simulink model "untitled"  (R2022b)
settings: Solver=VariableStepAuto  StartTime=0.0  StopTime=10.0  RelTol=1e-3
undefined symbols (not defined in the file): F, g, J, M, mass, quadrotor
libraries: slpidlib x4, simulink x2, matrix_library x1
settings Model: Creator=Musta  LastModifiedBy=Musta

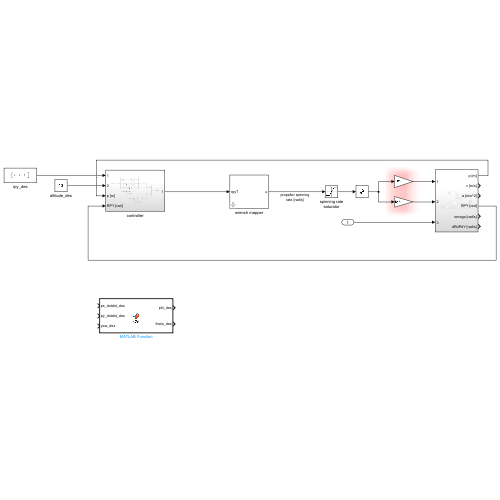
[thumbnail: Simulink's stored preview of the top-level diagram]
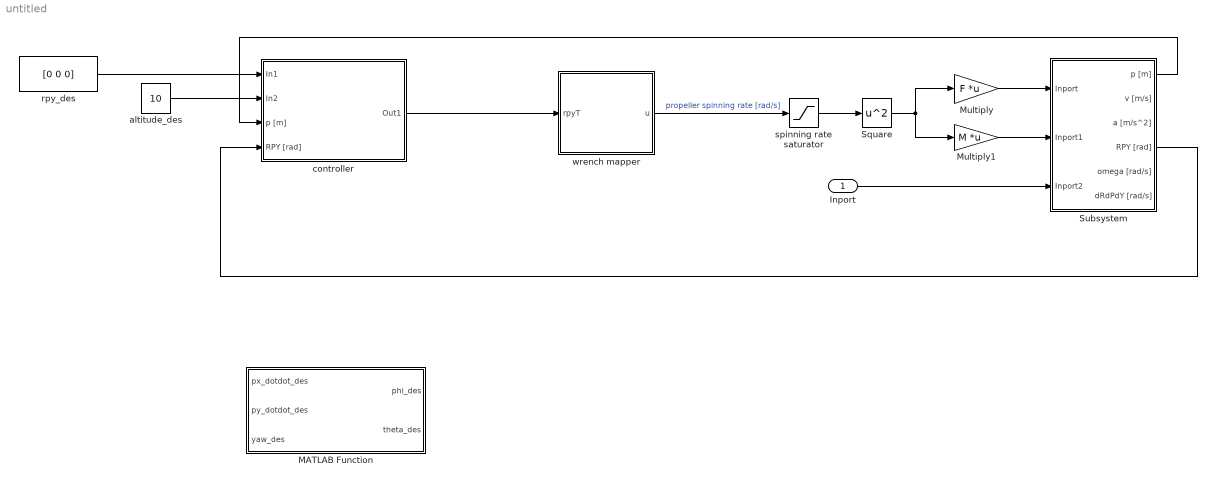
== system untitled ==
  Inport : Inport
  MATLAB Function : MATLAB Function  TreatAsAtomicUnit=on
  Multiply : Gain  Gain=F  Multiplication=Matrix(K*u)
  Multiply1 : Gain  Gain=M  Multiplication=Matrix(K*u)
  Square : Math  Operator=square
  Subsystem : Subsystem
  altitude_des : Constant  Value=10
  controller : Subsystem
  rpy_des : Constant  Value=[0 0 0]
  spinning rate saturator : Saturate
  wrench mapper : Subsystem  mask(wrench mapper){mapperMatrix=quadrotor.mixer.wrenchMapper}
      mask prompts: mapperMatrix "mapper matrix"
      mask help:
      | maps desired roll, pitch, yaw torque and total common thrust into the input vector u for a quadrotor.
      | input: [tau_roll, tau_pitch, tau_yaw, thrust]
      | input unit: [Nm, Nm, Nm, N]
      | output [u_1, u_2, u_3, u_3]
      | output unit: [rad^2/s^2]
      mask TypeOptions mapperMatrix: mapper/Gain
  wires:
  Multiply/1 -> Subsystem/1(Inport)
  Multiply1/1 -> Subsystem/2(Inport1)
  Inport/1 -> Subsystem/3(Inport2)
  Square/1 -> Multiply/1, Multiply1/1
  spinning rate saturator/1 -> Square/1
  wrench mapper/1(u) -> spinning rate saturator/1  "propeller spinning rate [rad/s]"
  Subsystem/1(p [m]) -> controller/3(p [m])
  controller/1(Out1) -> wrench mapper/1(rpyT)
  Subsystem/4(RPY [rad]) -> controller/4(RPY [rad])
  rpy_des/1 -> controller/1(In1)
  altitude_des/1 -> controller/2(In2)

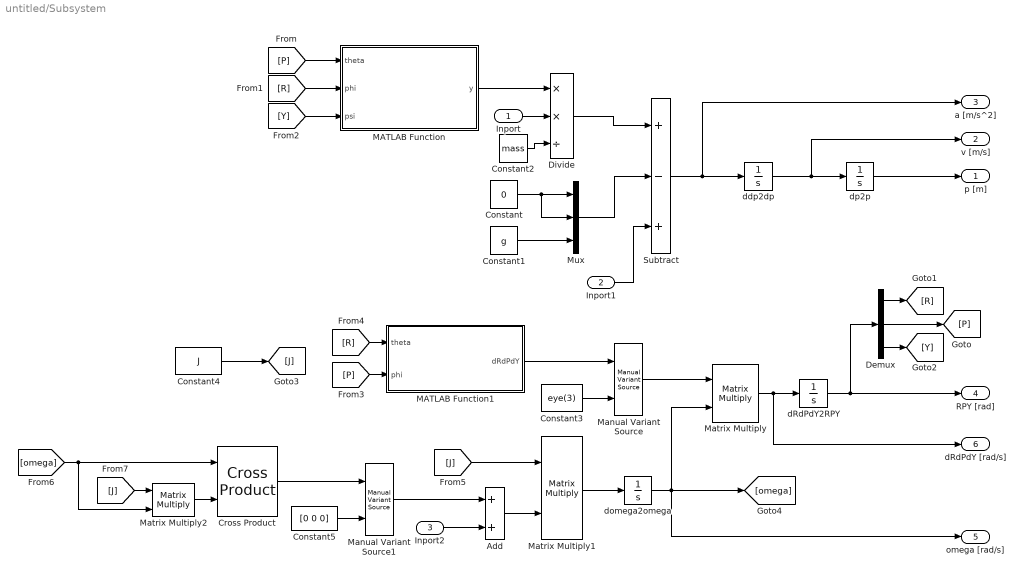
== system untitled/Subsystem ==
  Inport : Inport
  Inport1 : Inport  Port=2
  Inport2 : Inport  Port=3
  Add : Sum
  Constant : Constant  Value=0
  Constant1 : Constant  Value=g
  Constant2 : Constant  Value=mass
  Constant3 : Constant  Value=eye(3)
  Constant4 : Constant  Value=J
  Constant5 : Constant  Value=[0 0 0]
  Cross Product : matrix_library/Cross Product
  Demux : Demux  Outputs=3
  Divide : Product  Inputs=**/
  MATLAB Function : MATLAB Function  TreatAsAtomicUnit=on
  MATLAB Function1 : MATLAB Function  TreatAsAtomicUnit=on
  Manual Variant Source : simulink/Signal Routing/Manual Variant Source  NumChoices=2  LabelModeActiveChoice=V_1
  Manual Variant Source1 : simulink/Signal Routing/Manual Variant Source  NumChoices=2  LabelModeActiveChoice=V_1
  Matrix Multiply : Product  Multiplication=Matrix(*)
  Matrix Multiply1 : Product  Multiplication=Matrix(*)
  Matrix Multiply2 : Product  Multiplication=Matrix(*)
  Mux : Mux  Inputs=3
  Subtract : Sum  Inputs=+-+
  dRdPdY2RPY : Integrator
  ddp2dp : Integrator
  domega2omega : Integrator
  dp2p : Integrator
  p [m] : Outport
  v [m/s] : Outport  Port=2
  a [m/s^2] : Outport  Port=3
  RPY [rad] : Outport  Port=4
  omega [rad/s] : Outport  Port=5
  dRdPdY [rad/s] : Outport  Port=6
  wires:
  [R] -> MATLAB Function/2(phi)
  Inport2/1 -> Add/2
  ddp2dp/1 -> v [m/s]/1, dp2p/1
  Matrix Multiply/1 -> dRdPdY [rad/s]/1, dRdPdY2RPY/1
  MATLAB Function/1(y) -> Divide/1
  [R] -> MATLAB Function1/1(theta)
  Constant3/1 -> Manual Variant Source/2
  Inport1/1 -> Subtract/3
  domega2omega/1 -> omega [rad/s]/1, Matrix Multiply/2, [omega]
  [P] -> MATLAB Function/1(theta)
  Constant5/1 -> Manual Variant Source1/2
  Divide/1 -> Subtract/1
  [omega] -> Matrix Multiply2/2, Cross Product/1
  Constant2/1 -> Divide/3
  Inport/1 -> Divide/2
  Constant/1 -> Mux/2, Mux/1
  Mux/1 -> Subtract/2
  Matrix Multiply1/1 -> domega2omega/1
  Demux/2 -> [P]
  Add/1 -> Matrix Multiply1/2
  Manual Variant Source1/1 -> Add/1
  Manual Variant Source/1 -> Matrix Multiply/1
  MATLAB Function1/1(dRdPdY) -> Manual Variant Source/1
  dp2p/1 -> p [m]/1
  [P] -> MATLAB Function1/2(phi)
  Constant1/1 -> Mux/3
  Demux/1 -> [R]
  Subtract/1 -> a [m/s^2]/1, ddp2dp/1
  Demux/3 -> [Y]
  dRdPdY2RPY/1 -> RPY [rad]/1, Demux/1
  [J] -> Matrix Multiply2/1
  [Y] -> MATLAB Function/3(psi)
  Constant4/1 -> [J]
  Cross Product/1 -> Manual Variant Source1/1
  Matrix Multiply2/1 -> Cross Product/2
  [J] -> Matrix Multiply1/1

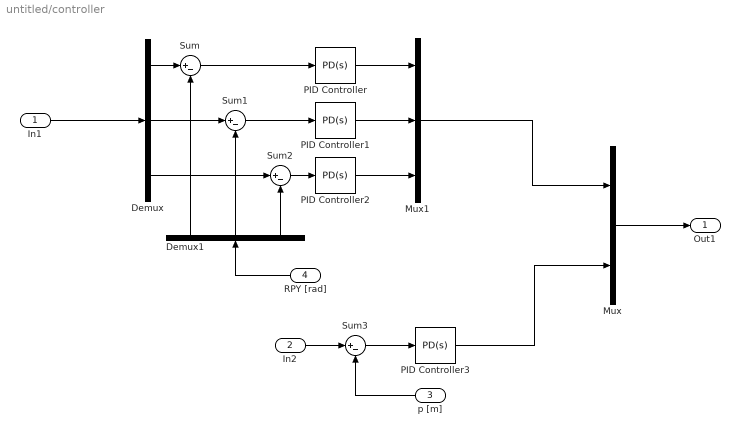
== system untitled/controller ==
  In1 : Inport
  In2 : Inport  Port=2
  p [m] : Inport  Port=3
  RPY [rad] : Inport  Port=4
  Demux : Demux  Outputs=3
  Demux1 : Demux  Outputs=3
  Mux : Mux  Inputs=2
  Mux1 : Mux  Inputs=3
  PID Controller{,1..3} (4 alike) : slpidlib/PID Controller  Controller=PD  Form=Parallel  TimeDomain=Continuous-time  UseExternalTs=off  SampleTime=-1  IntegratorMethod=Forward Euler  FilterMethod=Forward Euler  ControllerParametersSource=internal  P=1  I=1  UseKiTs=off  D=0  N=100  UseFilter=on  TunerSelectOption=Transfer Function Based (PID Tuner App)  InitialConditionSource=internal  InitialConditionForIntegrator=0  InitialConditionForFilter=0  DifferentiatorICPrevScaledInput=0  ExternalReset=none  TrackingMode=off  Kt=1  LimitOutput=off  SatLimitsSource=internal  UpperSaturationLimit=inf  LowerSaturationLimit=-inf  LinearizeAsGain=on  AntiWindupMode=none  Kb=1  LimitIntegrator=off  UpperIntegratorSaturationLimit=inf  LowerIntegratorSaturationLimit=-inf  POutMin=[]  POutMax=[]  IOutMin=[]  IOutMax=[]  DOutMin=[]  DOutMax=[]  NOutMin=[]  NOutMax=[]  SumOutMin=[]  SumOutMax=[]  SaturationOutMin=[]  SaturationOutMax=[]  PParamMin=[]  PParamMax=[]  IParamMin=[]  IParamMax=[]  DParamMin=[]  DParamMax=[]  NParamMin=[]  NParamMax=[]  KbParamMin=[]  KbParamMax=[]  KtParamMin=[]  KtParamMax=[]  KbOutMin=[]  KbOutMax=[]  KtOutMin=[]  KtOutMax=[]  IntegratorOutMin=[]  IntegratorOutMax=[]  FilterOutMin=[]  FilterOutMax=[]  SumI1OutMin=[]  SumI1OutMax=[]  SumI2OutMin=[]  SumI2OutMax=[]  SumI3OutMin=[]  SumI3OutMax=[]  SumI4OutMin=[]  SumI4OutMax=[]  SumDOutMin=[]  SumDOutMax=[]  DifferentiatorOutMin=[]  DifferentiatorOutMax=[]  FilterDiffOutCoefMin=[]  FilterDiffOutCoefMax=[]  ReciprocalOutMin=[]  ReciprocalOutMax=[]  SumDenOutMin=[]  SumDenOutMax=[]  SumNumOutMin=[]  SumNumOutMax=[]  DivideOutMin=[]  DivideOutMax=[]  UdiffTsProdOutMin=[]  UdiffTsProdOutMax=[]  NTsProdOutMin=[]  NTsProdOutMax=[]  UintegralTsProdOutMin=[]  UintegralTsProdOutMax=[]  UngainTsProdOutMin=[]  UngainTsProdOutMax=[]  ClampingZeroOutDataTypeStr=Inherit: Inherit via back propagation  ClampingZeroOutMin=[]  ClampingZeroOutMax=[]  FilterDenConstantOutDataTypeStr=Inherit: Inherit via back propagation  FilterDenConstantOutMin=[]  FilterDenConstantOutMax=[]  PCopyOutDataTypeStr=Inherit: Inherit via back propagation  PCopyOutMin=[]  PCopyOutMax=[]  NCopyOutDataTypeStr=Inherit: Inherit via back propagation  NCopyOutMin=[]  NCopyOutMax=[]  IntegratorContinuousStateAttributes=''  IntegratorStateMustResolveToSignalObject=off  IntegratorRTWStateStorageClass=Auto  FilterContinuousStateAttributes=''  FilterStateMustResolveToSignalObject=off  FilterRTWStateStorageClass=Auto  ParallelPVariant=InternalParameters  IdealPVariant=Disabled  IVariant=Disabled  DVariant=InternalParameters  IntegratorVariant=Disabled  SatVariant=Disabled  AWVariant=Disabled  PCopyVariant=Disabled  TRVariant=Disabled  FdbkBlocksVariant=Forward  IdealPFdbkVariant=Disabled  SatFdbkVariant=Disabled  DerivativeFilterVariant=ContFilter  NVariant=InternalParameters  NCopyVariant=Disabled  FilterICVariant=InternalICsFilter  IntegratorICVariant=Disabled  ExternalResetVariant=Disabled  TRSumVariant=Passthrough  SumFdbkVariant=Disabled  SumVariant=Sum_PD  TsampFilterVariant=InternalTs  TsampNgainVariant=Passthrough  TsampIntegralVariant=Disabled_SignalSpec  ExternalSaturationOutDataTypeStr=Inherit: Same as second input
  Sum{,1..3} (4 alike) : Sum  Inputs=|+-
  Out1 : Outport
  wires:
  Demux1/1 -> Sum/2
  Mux/1 -> Out1/1
  Demux/1 -> Sum/1
  PID Controller/1 -> Mux1/1
  Sum1/1 -> PID Controller1/1
  Mux1/1 -> Mux/1
  Sum/1 -> PID Controller/1
  Demux/2 -> Sum1/1
  PID Controller2/1 -> Mux1/3
  Sum2/1 -> PID Controller2/1
  Demux/3 -> Sum2/1
  Demux1/2 -> Sum1/2
  PID Controller3/1 -> Mux/2
  Sum3/1 -> PID Controller3/1
  Demux1/3 -> Sum2/2
  PID Controller1/1 -> Mux1/2
  RPY [rad]/1 -> Demux1/1
  In1/1 -> Demux/1
  p [m]/1 -> Sum3/2
  In2/1 -> Sum3/1

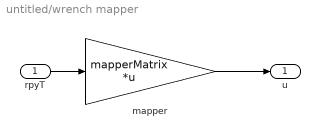
== system untitled/wrench mapper ==
  rpyT : Inport
  mapper : Gain  Gain=mapperMatrix  Multiplication=Matrix(K*u)
  u : Outport
  wires:
  mapper/1 -> u/1
  rpyT/1 -> mapper/1

== matlab function untitled/Subsystem/MATLAB Function1 ==
  data: theta input; dRdPdY output; phi input
function dRdPdY = fcn(theta, phi)

    

end

== matlab function untitled/Subsystem/MATLAB Function ==
  data: theta input; y output; phi input; psi input
function y = fcn(theta, phi, psi)

    

end

== matlab function untitled/MATLAB Function ==
  data: px_dotdot_des input; phi_des output; py_dotdot_des input; yaw_des input; theta_des output
function [phi_des, theta_des] = p2a(px_dotdot_des, py_dotdot_des, yaw_des)

    %#codegen
    coder.extrinsic('evalin')
    g = 0;                  % Needed in order to set variable class correctly
    g = evalin('base','g'); % Read value from workspace

    phi_des = 1/g * (px_dotdot_des*sin(yaw_des) - py_dotdot_des*cos(yaw_des));
    theta_des = 1/g * (px_dotdot_des*cos(yaw_des) + py_dotdot_des*sin(yaw_des));

end
